simulink model "abs_CS9_rlnonmoon"  (R2023a)
settings: Solver=ode45  StartTime=0  StopTime=10  FixedStep=0.002  RelTol=1e-3  AbsTol=1e-6
undefined symbols (not defined in the file or in its folder): DiscIntNeverNeededParam
libraries: simulink x3, Solver_SF x1, rllib x1
settings Model: ExtModeTrigMode=oneshot  Creator=ywata  LastModifiedBy=USER
settings SolverCC: AutoScaleAbsTol=off  AlgebraicLoopSolver=TrustRegion
settings DataIOCC: SaveFormat=Array  SignalLoggingSaveFormat=ModelDataLogs  ReturnWorkspaceOutputs=off  SignalLoggingName=sigsOut
settings OptimizationCC: BlockReduction=off  BooleanDataType=off  ExpressionDepthLimit=2147483647  LifeSpan=inf
settings DebuggingCC: SaveWithParameterizedLinksMsg=none  UnderspecifiedInitializationDetection=Classic  MergeDetectMultiDrivingBlocksExec=none  SignalResolutionControl=TryResolveAllWithWarning  MultiTaskDSMMsg=warning  MultiTaskCondExecSysMsg=none  FcnCallInpInsideContextMsg=warning  UnconnectedInputMsg=warning  UnconnectedOutputMsg=warning  UnconnectedLineMsg=warning  StateNameClashWarn=warning  SFUnexpectedBacktrackingDiag=warning  SFNoUnconditionalDefaultTransitionDiag=warning  SFExecutionAtInitializationDiag=none  ArithmeticOperatorsInVariantConditions=warning
settings HardwareCC: ProdBitPerPointer=32  ProdBitPerSizeT=32  ProdBitPerPtrDiffT=32  ProdLargestAtomicFloat=None  ProdIntDivRoundTo=Undefined  ProdEndianess=Unspecified  ProdWordSize=32  ProdHWDeviceType=32-bit Generic  TargetUnknown=on
settings ModelReferenceCC: PropagateSignalLabelsOutOfModel=off
settings SFSimCC: SimUseLocalCustomCode=off  CustomCodeUndefinedFunction=UseInterfaceOnly
settings RTWCC: TemplateMakefile=grt_vc.tmf  RTWUseLocalCustomCode=off
settings CodeAppCC: StateflowObjectComments=on
settings GRTTargetCC: TargetFcnLib=ansi_tfl_tmw.mat  TargetLangStandard=C89/C90 (ANSI)  CombineOutputUpdateFcns=off  GRTInterface=on
settings ConfigComp: CovMetricSettings=dw  CovSaveCumulativeToWorkspaceVar=on  CovSaveSingleToWorkspaceVar=on  CovExternalEMLEnable=off

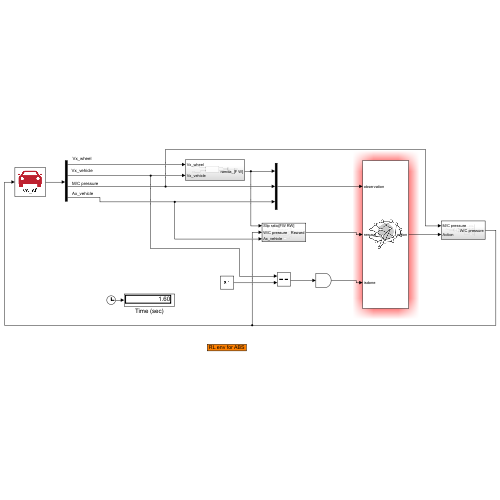
[thumbnail: Simulink's stored preview of the top-level diagram]
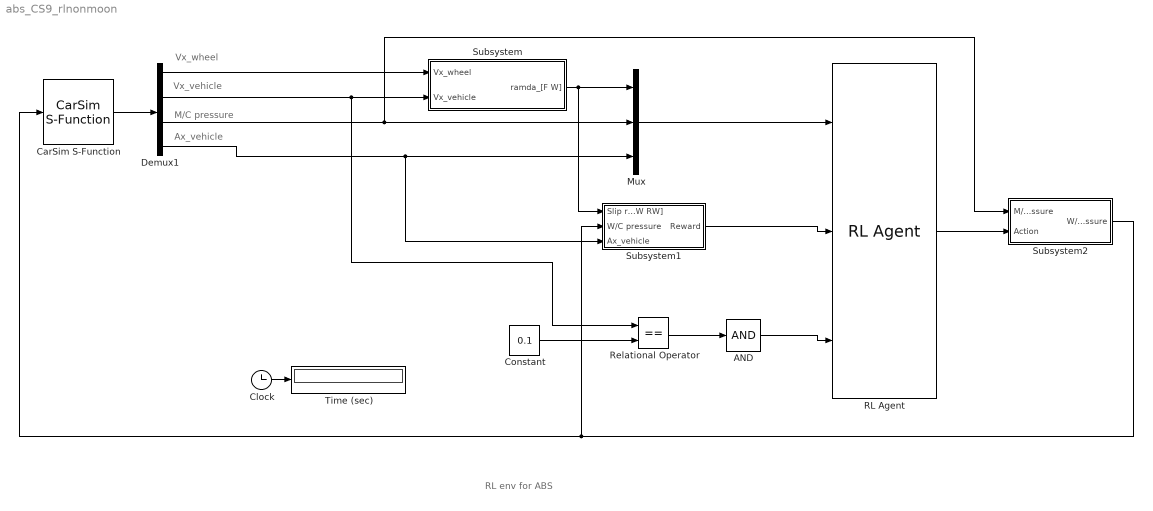
== system abs_CS9_rlnonmoon ==
  note: Ax_vehicle
  note: M/C pressure
  note: Vx_vehicle
  note: Vx_wheel
  note: RL env for ABS
  AND : Logic  Inputs=1  IconShape=distinctive  AllPortsSameDT=off  OutDataTypeStr=boolean
  CarSim S-Function : Solver_SF/CarSim S-Function  Priority=1  SIMFILE=simfile.sim  Run_RTs=off  vs_state_ind=Run  StopMode_ind=Vehicle Model
  Clock : Clock
  Constant : Constant  Value=0.1
  Demux1 : Demux  Outputs=[4 1 1 1]
      settings: DisplayOption=none
  Mux : Mux  Inputs=[2 1 1]
  RL Agent : rllib/RL Agent  Agent=agentObj  ExternalActionAsInput=off  ProvideLastAction=off  ProvideCumRwd=off  TreatAsDirectFeedthrough=on  UseStrictObservationDataTypes=off
  Relational Operator : RelationalOperator  Operator===  OutDataTypeStr=boolean  RndMeth=Simplest  InputSameDT=off
  Subsystem : Subsystem
  Subsystem1 : Subsystem
  Subsystem2 : Subsystem
  Time (sec) : Display
      settings: Format=bank  Decimation=100
  wires:
  CarSim S-Function/1 -> Demux1/1
  Demux1/2 -> Relational Operator/1, Subsystem/2(Vx_vehicle)
  Demux1/1 -> Subsystem/1(Vx_wheel)
  Clock/1 -> Time (sec)/1
  Demux1/3 -> Subsystem2/1(M/C pressure), Mux/2
  Demux1/4 -> Subsystem1/3(Ax_vehicle), Mux/3
  Subsystem/1(ramda_[F W]) -> Subsystem1/1(Slip ratio[FW RW]), Mux/1
  Mux/1 -> RL Agent/1
  Subsystem1/1(Reward) -> RL Agent/2
  AND/1 -> RL Agent/3
  Relational Operator/1 -> AND/1
  Constant/1 -> Relational Operator/2
  RL Agent/1 -> Subsystem2/2(Action)
  Subsystem2/1(W/C pressure) -> Subsystem1/2(W/C pressure), CarSim S-Function/1

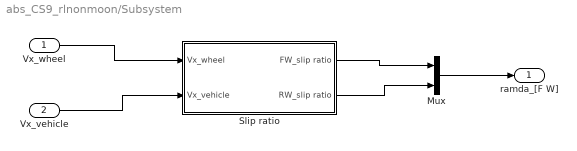
== system abs_CS9_rlnonmoon/Subsystem ==
  Vx_wheel : Inport
  Vx_vehicle : Inport  Port=2
  Mux : Mux  Inputs=2
  Slip ratio : Subsystem
  ramda_[F W] : Outport
  wires:
  Vx_wheel/1 -> Slip ratio/1(Vx_wheel)
  Vx_vehicle/1 -> Slip ratio/2(Vx_vehicle)
  Slip ratio/1(FW_slip ratio) -> Mux/1
  Slip ratio/2(RW_slip ratio) -> Mux/2
  Mux/1 -> ramda_[F W]/1

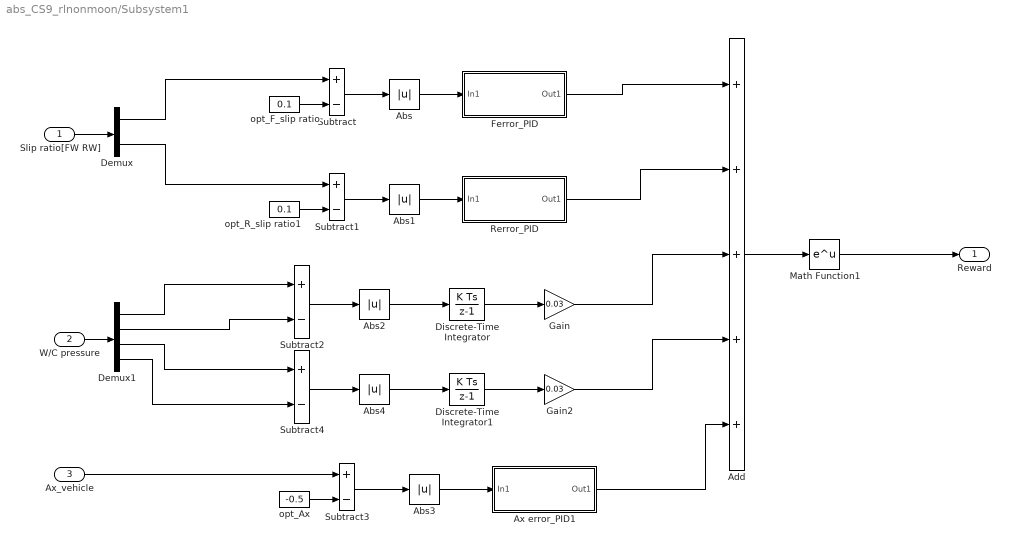
== system abs_CS9_rlnonmoon/Subsystem1 ==
  Slip ratio[FW RW] : Inport
  W/C pressure : Inport  Port=2
  Ax_vehicle : Inport  Port=3
  Abs{,1..4} (5 alike) : Abs  SaturateOnIntegerOverflow=off
  Add : Sum  Inputs=+++++
  Ax error_PID1 : Subsystem
  Demux : Demux  Outputs=2
  Demux1 : Demux
  Discrete-Time Integrator : DiscreteIntegrator  SampleTime=-1  ICPrevOutput=DiscIntNeverNeededParam  ICPrevScaledInput=DiscIntNeverNeededParam
  Discrete-Time Integrator1 : DiscreteIntegrator  SampleTime=-1  ICPrevOutput=DiscIntNeverNeededParam  ICPrevScaledInput=DiscIntNeverNeededParam
  Ferror_PID : Subsystem
  Gain : Gain  Gain=0.03
  Gain2 : Gain  Gain=0.03
  Math Function1 : Math
  Rerror_PID : Subsystem
  Subtract{,1..4} (5 alike) : Sum  Inputs=+-
  opt_Ax : Constant  Value=-0.5
  opt_F_slip ratio : Constant  Value=0.1
  opt_R_slip ratio1 : Constant  Value=0.1
  Reward : Outport
  wires:
  Slip ratio[FW RW]/1 -> Demux/1
  Demux/1 -> Subtract/1
  Demux/2 -> Subtract1/1
  opt_F_slip ratio/1 -> Subtract/2
  opt_R_slip ratio1/1 -> Subtract1/2
  Subtract/1 -> Abs/1
  Subtract1/1 -> Abs1/1
  Abs/1 -> Ferror_PID/1(In1)
  Abs1/1 -> Rerror_PID/1(In1)
  Ferror_PID/1(Out1) -> Add/1
  Rerror_PID/1(Out1) -> Add/2
  Subtract2/1 -> Abs2/1
  Abs2/1 -> Discrete-Time Integrator/1
  Discrete-Time Integrator/1 -> Gain/1
  Ax_vehicle/1 -> Subtract3/1
  opt_Ax/1 -> Subtract3/2
  Subtract3/1 -> Abs3/1
  Abs3/1 -> Ax error_PID1/1(In1)
  Ax error_PID1/1(Out1) -> Add/5
  Add/1 -> Math Function1/1
  Math Function1/1 -> Reward/1
  W/C pressure/1 -> Demux1/1
  Discrete-Time Integrator1/1 -> Gain2/1
  Abs4/1 -> Discrete-Time Integrator1/1
  Demux1/4 -> Subtract4/2
  Subtract4/1 -> Abs4/1
  Demux1/1 -> Subtract2/1
  Demux1/3 -> Subtract4/1
  Gain/1 -> Add/3
  Gain2/1 -> Add/4
  Demux1/2 -> Subtract2/2

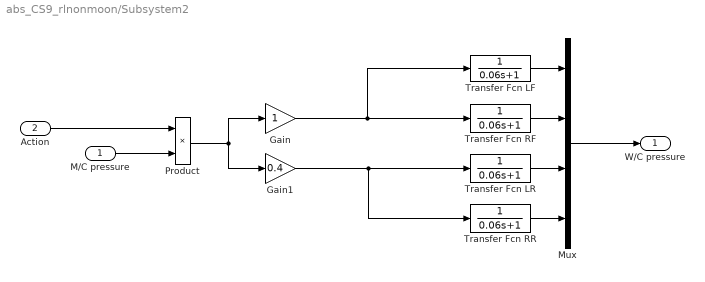
== system abs_CS9_rlnonmoon/Subsystem2 ==
  M/C pressure : Inport
  Action : Inport  Port=2
  Gain : Gain
  Gain1 : Gain  Gain=0.4
  Mux : Mux
  Product : Product
  Transfer Fcn LF : TransferFcn  Denominator=[0.06 1]
  Transfer Fcn LR : TransferFcn  Denominator=[0.06 1]
  Transfer Fcn RF : TransferFcn  Denominator=[0.06 1]
  Transfer Fcn RR : TransferFcn  Denominator=[0.06 1]
  W/C pressure : Outport
  wires:
  Action/1 -> Product/1
  M/C pressure/1 -> Product/2
  Product/1 -> Gain1/1, Gain/1
  Gain/1 -> Transfer Fcn LF/1, Transfer Fcn RF/1
  Gain1/1 -> Transfer Fcn RR/1, Transfer Fcn LR/1
  Transfer Fcn LF/1 -> Mux/1
  Transfer Fcn RF/1 -> Mux/2
  Transfer Fcn LR/1 -> Mux/3
  Transfer Fcn RR/1 -> Mux/4
  Mux/1 -> W/C pressure/1

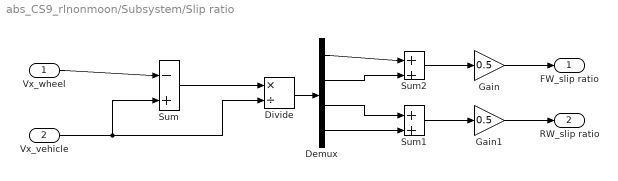
== system abs_CS9_rlnonmoon/Subsystem/Slip ratio ==
  Vx_wheel : Inport
  Vx_vehicle : Inport  Port=2
  Demux : Demux
  Divide : Product  Inputs=*/
  Gain : Gain  Gain=0.5
  Gain1 : Gain  Gain=0.5
  Sum : Sum  Inputs=-|+
  Sum1 : Sum  Inputs=+|+
  Sum2 : Sum  Inputs=+|+
  FW_slip ratio : Outport
  RW_slip ratio : Outport  Port=2
  wires:
  Vx_wheel/1 -> Sum/1
  Vx_vehicle/1 -> Divide/2, Sum/2
  Sum/1 -> Divide/1
  Divide/1 -> Demux/1
  Demux/1 -> Sum2/1
  Demux/2 -> Sum2/2
  Demux/4 -> Sum1/2
  Demux/3 -> Sum1/1
  Sum2/1 -> Gain/1
  Sum1/1 -> Gain1/1
  Gain/1 -> FW_slip ratio/1
  Gain1/1 -> RW_slip ratio/1

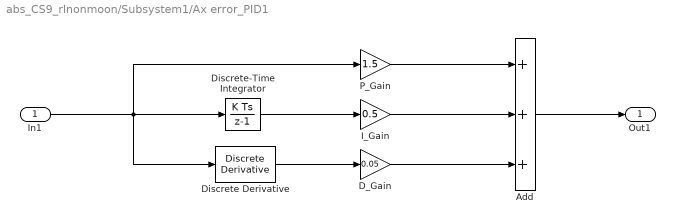
== system abs_CS9_rlnonmoon/Subsystem1/Ax error_PID1 ==
  In1 : Inport
  Add : Sum  Inputs=+++
  D_Gain : Gain  Gain=0.05
  Discrete Derivative : simulink/Discrete/Discrete Derivative  gainval=1.0  ICPrevScaledInput=0.0  OutMin=[]  OutMax=[]  OutDataType=fixdt(1, 16)  OutScaling=2^-10  DoSatur=off
  Discrete-Time Integrator : DiscreteIntegrator  SampleTime=-1  ICPrevOutput=DiscIntNeverNeededParam  ICPrevScaledInput=DiscIntNeverNeededParam
  I_Gain : Gain  Gain=0.5
  P_Gain : Gain  Gain=1.5
  Out1 : Outport
  wires:
  Add/1 -> Out1/1
  In1/1 -> P_Gain/1, Discrete-Time Integrator/1, Discrete Derivative/1
  Discrete Derivative/1 -> D_Gain/1
  D_Gain/1 -> Add/3
  Discrete-Time Integrator/1 -> I_Gain/1
  I_Gain/1 -> Add/2
  P_Gain/1 -> Add/1

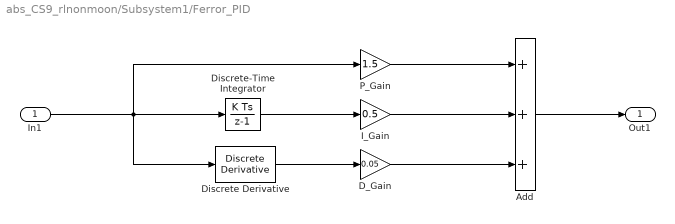
== system abs_CS9_rlnonmoon/Subsystem1/Ferror_PID ==
  In1 : Inport
  Add : Sum  Inputs=+++
  D_Gain : Gain  Gain=0.05
  Discrete Derivative : simulink/Discrete/Discrete Derivative  gainval=1.0  ICPrevScaledInput=0.0  OutMin=[]  OutMax=[]  OutDataType=fixdt(1, 16)  OutScaling=2^-10  DoSatur=off
  Discrete-Time Integrator : DiscreteIntegrator  SampleTime=-1  ICPrevOutput=DiscIntNeverNeededParam  ICPrevScaledInput=DiscIntNeverNeededParam
  I_Gain : Gain  Gain=0.5
  P_Gain : Gain  Gain=1.5
  Out1 : Outport
  wires:
  Add/1 -> Out1/1
  In1/1 -> P_Gain/1, Discrete-Time Integrator/1, Discrete Derivative/1
  Discrete Derivative/1 -> D_Gain/1
  D_Gain/1 -> Add/3
  Discrete-Time Integrator/1 -> I_Gain/1
  I_Gain/1 -> Add/2
  P_Gain/1 -> Add/1

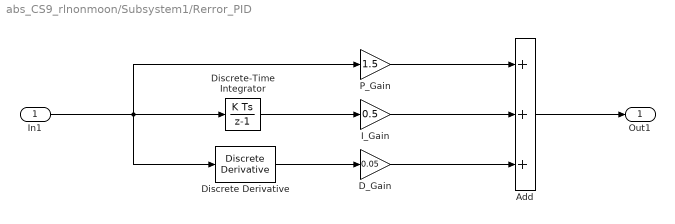
== system abs_CS9_rlnonmoon/Subsystem1/Rerror_PID ==
  In1 : Inport
  Add : Sum  Inputs=+++
  D_Gain : Gain  Gain=0.05
  Discrete Derivative : simulink/Discrete/Discrete Derivative  gainval=1.0  ICPrevScaledInput=0.0  OutMin=[]  OutMax=[]  OutDataType=fixdt(1, 16)  OutScaling=2^-10  DoSatur=off
  Discrete-Time Integrator : DiscreteIntegrator  SampleTime=-1  ICPrevOutput=DiscIntNeverNeededParam  ICPrevScaledInput=DiscIntNeverNeededParam
  I_Gain : Gain  Gain=0.5
  P_Gain : Gain  Gain=1.5
  Out1 : Outport
  wires:
  Add/1 -> Out1/1
  In1/1 -> P_Gain/1, Discrete-Time Integrator/1, Discrete Derivative/1
  Discrete Derivative/1 -> D_Gain/1
  D_Gain/1 -> Add/3
  Discrete-Time Integrator/1 -> I_Gain/1
  I_Gain/1 -> Add/2
  P_Gain/1 -> Add/1
